simulink model "sim_ff_velocity"  (R2022a)
settings: Solver=FixedStepAuto  StartTime=0.0  StopTime=120  FixedStep=1e-2  RelTol=1e-3
values from neighbouring files (symbols this model uses):
  b = 226    [simulateModel.m]
  cm = 2    [simulateModel.m]
  ct = 1    [simulateModel.m]
  g = 9.81    [simulateModel.m]
  L = 1    [simulateModel.m]
  m = 75    [simulateModel.m]
  mns = randi(1e5,1)    [simulateModel.m]
  n_gain = 7    [simulateModel.m]
  nns = randi(1e5,1)    [simulateModel.m]
  wref = 5*(2*pi)/60    (= 0.523598775598)    [simulateModel.m]
libraries: simulink x4
settings Model: Creator=chopp  LastModifiedBy=rika

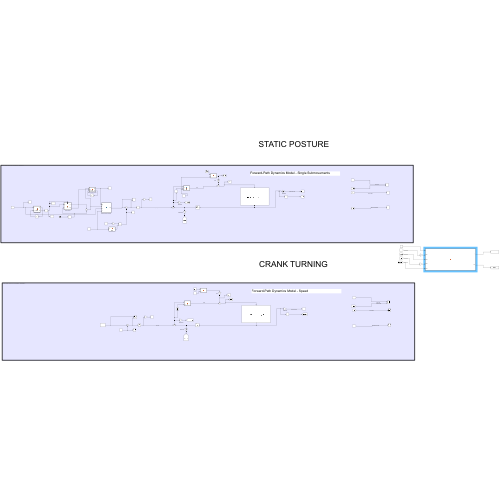
[thumbnail: Simulink's stored preview of the top-level diagram]
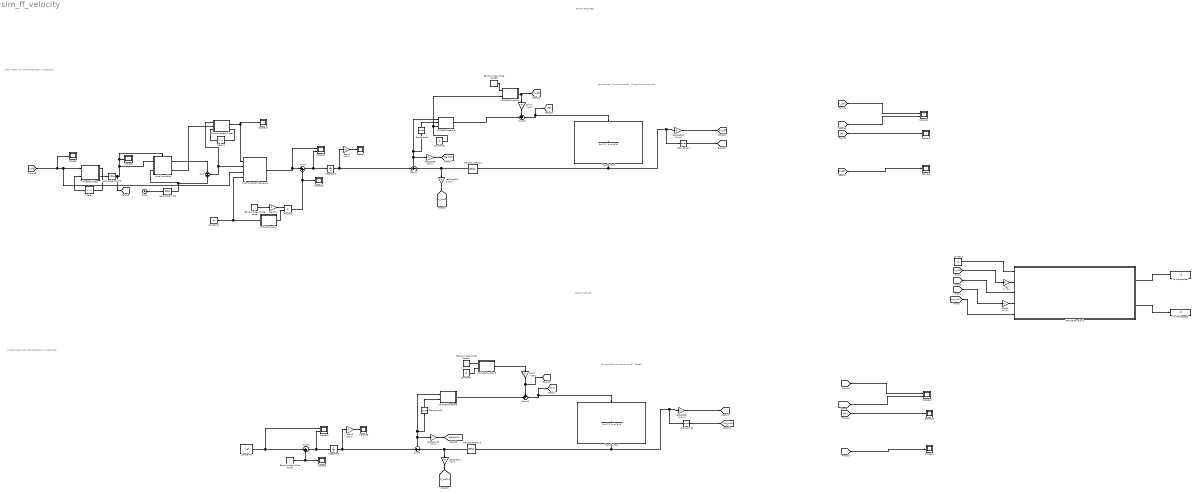
== system sim_ff_velocity ==
  note: STATIC POSTURE
  note: Forward-Path Dynamics Model - Single Submovements
  note: Linear Model with pole cancellation (-20db/dec)
  note: Linear Model with pole cancellation (-20db/dec)
  note: Forward-Path Dynamics Model - Speed
  note: CRANK TURNING
  Band-Limited White Noise : simulink/Sources/Band-Limited White Noise  Cov=[0.1]  Ts=0.08  seed=[nns]
  Band-Limited White Noise4 : simulink/Sources/Band-Limited White Noise  Cov=[0.0005]  Ts=0.08  seed=[nns]
  Band-Limited White Noise5 : simulink/Sources/Band-Limited White Noise  Cov=[0.1]  Ts=0.08  seed=[mns]
  Band-Limited White Noise9 : simulink/Sources/Band-Limited White Noise  Cov=[0.1]  Ts=0.08  seed=[mns]
  Clock : Clock
  Constant : Constant  Value=cm
  Constant1 : Constant  Value=ct
  Constant5 : Constant  Value=ct
  Constant7 : Constant  Value=ct
  Constant9 : Constant  Value=wref
  Delay : Delay  DelayLength=1
  Delay1 : Delay  DelayLength=1
  Derivative{4..5,9..10} (4 alike) : Derivative
  Gain : Gain  Gain=pi/180
  Gain1 : Gain  Gain=pi/180
  Gain10 : Gain
  Gain3 : Gain  Gain=180/pi
  Gain6 : Gain  Gain=180/pi
  Initial condition : MATLAB Function  TreatAsAtomicUnit=on
  Integrator1 : Integrator
  Integrator2 : Integrator
  MATLAB Function : MATLAB Function  TreatAsAtomicUnit=on
  MATLAB Function1 : MATLAB Function  TreatAsAtomicUnit=on
  MATLAB Function3 : MATLAB Function  TreatAsAtomicUnit=on
  MATLAB Function4 : MATLAB Function  TreatAsAtomicUnit=on
  MATLAB Function5 : MATLAB Function  TreatAsAtomicUnit=on
  MATLAB Function6 : MATLAB Function  TreatAsAtomicUnit=on
  Product : Product
  Scope{6..10,13,15..16,23..24,26} (11 alike) : Scope
  Scope{12,14,20,22} (4 alike) : Scope  NumInputPorts=2
  Submovement Generator : MATLAB Function  TreatAsAtomicUnit=on
  Submovement Timer : MATLAB Function  TreatAsAtomicUnit=on
  Sum : Sum  Inputs=-|+
  Sum10 : Sum  Inputs=++|
  Sum11 : Sum  Inputs=|++
  Sum12 : Sum  Inputs=+|-
  Sum13 : Sum  Inputs=++|
  Sum6 : Sum  Inputs=+|-
  Sum9 : Sum  Inputs=|++
  Threshold Flag : MATLAB Function  TreatAsAtomicUnit=on
  To Workspace1 : ToWorkspace  VariableName=x3  SaveFormat=Timeseries  SampleTime=-1
  To Workspace3 : ToWorkspace  VariableName=v3  SaveFormat=Timeseries  SampleTime=-1
  Transfer Fcn3 : TransferFcn  Denominator="[m*L^2  b -m*g*L]"
  Transfer Fcn4 : TransferFcn  Denominator="[m*L^2  b -m*g*L]"
  Transport Delay2 : TransportDelay  DelayTime=0.1
  Transport Delay5 : TransportDelay  DelayTime=0.1
  Zero-Order Hold : ZeroOrderHold  SampleTime=-1
  Zero-Order Hold3 : ZeroOrderHold  SampleTime=-1
  gain1 : Gain  Gain=n_gain
  gain2 : Gain  Gain=n_gain
  rad2grad{6,9..12,15} (6 alike) : Gain  Gain=180/pi
  wires:
  Initial condition/2(flag) -> Submovement Timer/2(flag)
  Gain6/1 -> Scope7/1
  Band-Limited White Noise/1 -> Gain10/1
  Sum/1 -> Submovement Timer/1(t), Submovement Generator/2(t)
  Submovement Timer/1(trig) -> Scope13/1, Submovement Generator/1(trig)
  Submovement Timer/2(idx) -> Delay1/1
  Delay1/1 -> Submovement Timer/3(idx_out)
  Integrator1/1 -> Gain6/1, Sum12/1  "x0 [rad]"
  Zero-Order Hold/1 -> Initial condition/2(t), Sum/2
  Sum9/1 -> Scope12/2, Integrator1/1
  Threshold Flag/1(thr) -> Delay/1
  Threshold Flag/2(fire) -> Zero-Order Hold3/1
  Delay/1 -> Threshold Flag/2(thr_old)
  Initial condition/1(t_tr) -> Sum/1
  [x_m3] -> Scope6/1, Submovement Generator/3(th), Threshold Flag/1(th)
  Zero-Order Hold3/1 -> [int_idx3], Initial condition/1(fire), Initial condition/Trigger, Scope9/1
  Submovement Generator/1(xd0) -> Scope12/1, Sum9/1
  Clock/1 -> Zero-Order Hold/1
  rad2grad9/1 -> [DeltaX3]
  Sum12/1 -> Derivative5/1, MATLAB Function5/1(u), rad2grad9/1
  [n_d3] -> Scope16/1  "External Noise [Nm]"
  Derivative5/1 -> MATLAB Function5/2(ud)
  Constant5/1 -> MATLAB Function4/2(ct), MATLAB Function5/3(ct)
  MATLAB Function4/1(y) -> [n_d3], gain1/1  "external disturbance"
  rad2grad10/1 -> [x_m3]  "Ankle Angle [deg]"
  [F3] -> Scope15/1  "Torque [Nm]"
  Sum13/1 -> [F3], Transfer Fcn3/1
  Derivative4/1 -> [xd_m3]
  [int_idx3] -> Scope14/2  "Control Switch"
  MATLAB Function5/1(y) -> Sum13/2  "torque"
  Band-Limited White Noise9/1 -> MATLAB Function4/1(u)
  [x_m3] -> Scope14/1  "Angle [deg]"
  Transfer Fcn3/1 -> Transport Delay2/1, Derivative4/1, rad2grad10/1  "angle"
  rad2grad12/1 -> [x_mn3]
  Product/1 -> Scope10/1, Sum9/2
  gain1/1 -> Sum13/1
  [n_d3v] -> Scope24/1  "External Noise [Nm]"
  Constant7/1 -> MATLAB Function3/2(ct)
  Derivative9/1 -> [xd_m3v]
  MATLAB Function3/1(y) -> gain2/1  "external disturbance"
  Derivative10/1 -> MATLAB Function6/2(ud)
  Transfer Fcn4/1 -> Transport Delay5/1, Derivative9/1, rad2grad6/1  "angle"
  [int_idx3v] -> Scope22/2  "Control Switch"
  Sum10/1 -> [F3v], Transfer Fcn4/1
  Sum6/1 -> Derivative10/1, MATLAB Function6/1(u), rad2grad15/1
  rad2grad15/1 -> [DeltaX3v]
  [x_m3v] -> Scope22/1  "Angle [deg]"
  Integrator2/1 -> Gain3/1, Sum6/1  "x0 [rad]"
  Sum11/1 -> Scope20/2, Integrator2/1
  [F3v] -> Scope23/1  "Torque [Nm]"
  Gain3/1 -> Scope26/1
  Band-Limited White Noise4/1 -> Scope8/1, Sum11/2
  Band-Limited White Noise5/1 -> MATLAB Function3/1(u)
  rad2grad6/1 -> [x_m3v]  "Ankle Angle [deg]"
  gain2/1 -> [n_d3v], Sum10/1
  rad2grad11/1 -> [x_mn3v]
  MATLAB Function6/1(y) -> Sum10/2  "torque"
  Constant9/1 -> Scope20/1, Sum11/1
  Transport Delay2/1 -> rad2grad12/1, Sum12/2
  Transport Delay5/1 -> rad2grad11/1, Sum6/2
  Constant1/1 -> Submovement Generator/4(ct), MATLAB Function/1(ct)
  MATLAB Function/1(y) -> Product/2
  Gain10/1 -> Product/1
  MATLAB Function1/1(y) -> To Workspace1/1
  MATLAB Function1/2(yd) -> To Workspace3/1
  Constant/1 -> MATLAB Function1/1(cm)
  [x_m3] -> Gain/1  "Angle [deg]"
  [xd_m3] -> MATLAB Function1/3(xd)  "Angle [deg]"
  [x_m3v] -> Gain1/1  "Angle [deg]"
  [xd_m3v] -> MATLAB Function1/5(xdv)  "Angle [deg]"
  Gain/1 -> MATLAB Function1/2(x)
  Gain1/1 -> MATLAB Function1/4(xv)

== matlab function sim_ff_velocity/MATLAB Function1 ==
  data: cm input; y output; yd output; x input; xd input; xv input; xdv input
function [y,yd] = fcn(cm, x, xd, xv, xdv)

if cm == 1
    y = x;
    yd = xd;
else
    y = xv;
    yd = xdv;
end

== matlab function sim_ff_velocity/MATLAB Function ==
  data: ct input; y output
function y = fcn(ct)

if ct == 1
    y = 0.001;
else
    y = 0.01;
end

== matlab function sim_ff_velocity/Initial condition ==
  data: fire input; t_tr output; t input; flag output
  events: trigger input RISING_EDGE_EVENT
function [t_tr,flag]  = fcn(fire, t)

t_tr = t*fire;
flag = 1;

end

== matlab function sim_ff_velocity/Submovement Generator ==
  data: trig input; xd0 output; t input; th input; ct input
function xd0 = fcn(trig, t, th, ct)
if ct == 1
    % Inverted Pendulum
    a = 0.015; %[rad/s]
else
    % Planar Roboti Link
    a = 0.120; %[rad/s]
end

b = 0.125; %[s]
c = 0.03; %[s]

sgn = -sign(th);

if trig == 0.2
    xd0 = sgn*a*exp(-((t-b)^2)/(2*c^2));
else 
    xd0 = 0;
end

end

== matlab function sim_ff_velocity/Submovement Timer ==
  data: t input; flag input; trig output; idx output; idx_out input
function [trig,idx] = fcn(t, flag, idx_out)

idx = idx_out+1;

if (t == 0 && flag == 1)
    idx = 0;
else
    idx = idx;
end

if (idx <= 20 && flag == 1)
    trig = 0.2;
else
    trig = 0;
end

end

== matlab function sim_ff_velocity/Threshold Flag ==
  data: th input; thr output; thr_old input; fire output
function [thr,fire]  = fcn(th, thr_old)

if (abs(th) > 2)
    thr = 1;
else
    thr = 0;
end

if (thr-thr_old) == 1
    fire = 1;
else
    fire = 0;
end

end

== matlab function sim_ff_velocity/MATLAB Function4 ==
  data: u input; y output; ct input
function y = fcn(u, ct)

if ct == 1
    y = u;
else
    y = 0.25*u;
end

== matlab function sim_ff_velocity/MATLAB Function5 ==
  data: u input; ud input; y output; ct input
function y  = fcn(u, ud, ct)

if ct == 1
    k = 1.2*75*9.81;
    b = 0*188.25;
else
    k = 65;
    b = 0;
end

y = k*u+b*ud;

end

== matlab function sim_ff_velocity/MATLAB Function3 ==
  data: u input; y output; ct input
function y = fcn(u, ct)

if ct == 1
    y = u;
else
    y = 0.25*u;
end

== matlab function sim_ff_velocity/MATLAB Function6 ==
  data: u input; ud input; y output
function y  = fcn(u, ud)

k = 65;
b = 0;

y = k*u+ b*ud;


end
